simulink model "simulacia_zadanie"  (R2019b)
settings: Solver=VariableStepAuto  StartTime=0.0  StopTime=0.25  RelTol=1e-3
values from neighbouring files (symbols this model uses):
  B = 0    [poit8.m]
  J = 0.85e-04    (= 8.5e-05)    [poit8.m]
  Kp = 1/30*(3*pi*J*Td*w0^2-pi*B)    (= 0.0014835298642)    [poit8.m]
  s1 = serial('COM141','BaudRate', 9600)    [poit8.m]
  SetPoint = double(output)    [poit8.m]
  Ti = (30*Kp)/(pi*J*w0^3*Td)    (= 0.018)    [poit8.m]
  w1 = 1/Ti    (= 55.5555555556)    [poit8.m]
  w2 = 1000    [poit8.m]
  xi1 = 1    [poit8.m]
  xi2 = 1    [poit8.m]
libraries: simulink x1
settings Model: Creator=ChosenOneX  LastModifiedBy=ChosenOneX

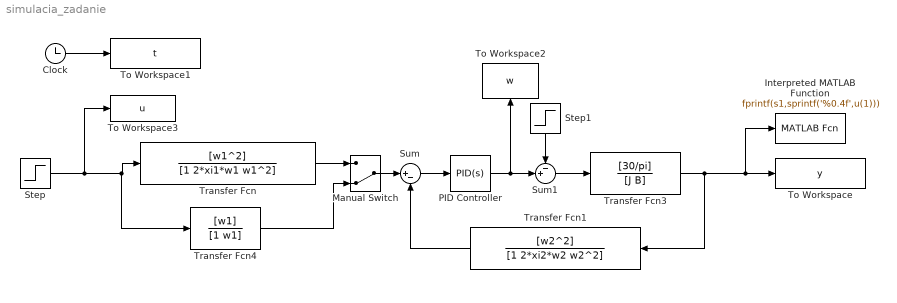
== system simulacia_zadanie ==
  Clock : Clock
  Interpreted MATLAB Function : MATLABFcn  MATLABFcn=fprintf(s1,sprintf('%0.4f',u(1)))  OutputDimensions=0
  Manual Switch : ManualSwitch  CurrentSetting=0
  PID Controller : simulink/Continuous/PID Controller  Controller=PID  Form=Parallel  TimeDomain=Continuous-time  SampleTime=-1  IntegratorMethod=Forward Euler  FilterMethod=Forward Euler  ControllerParametersSource=internal  P=Kp  I=Kp/Ti  D=0  UseFilter=on  N=100  TunerSelectOption=Transfer Function Based (PID Tuner App)  InitialConditionSource=internal  InitialConditionForIntegrator=0  InitialConditionForFilter=0  DifferentiatorICPrevScaledInput=0  ExternalReset=none  TrackingMode=off  Kt=1  LimitOutput=on  UpperSaturationLimit=7  LowerSaturationLimit=-7  LinearizeAsGain=on  AntiWindupMode=back-calculation  Kb=100  POutMin=[]  POutMax=[]  IOutMin=[]  IOutMax=[]  DOutMin=[]  DOutMax=[]  NOutMin=[]  NOutMax=[]  SumOutMin=[]  SumOutMax=[]  SaturationOutMin=[]  SaturationOutMax=[]  PParamMin=[]  PParamMax=[]  IParamMin=[]  IParamMax=[]  DParamMin=[]  DParamMax=[]  NParamMin=[]  NParamMax=[]  KbParamMin=[]  KbParamMax=[]  KtParamMin=[]  KtParamMax=[]  KbOutMin=[]  KbOutMax=[]  KtOutMin=[]  KtOutMax=[]  IntegratorOutMin=[]  IntegratorOutMax=[]  FilterOutMin=[]  FilterOutMax=[]  SumI1OutMin=[]  SumI1OutMax=[]  SumI2OutMin=[]  SumI2OutMax=[]  SumI3OutMin=[]  SumI3OutMax=[]  SumI4OutMin=[]  SumI4OutMax=[]  SumDOutMin=[]  SumDOutMax=[]  DifferentiatorOutMin=[]  DifferentiatorOutMax=[]  FilterDiffOutCoefMin=[]  FilterDiffOutCoefMax=[]  ReciprocalOutMin=[]  ReciprocalOutMax=[]  SumDenOutMin=[]  SumDenOutMax=[]  SumNumOutMin=[]  SumNumOutMax=[]  DivideOutMin=[]  DivideOutMax=[]  IntegratorContinuousStateAttributes=''  IntegratorStateMustResolveToSignalObject=off  IntegratorRTWStateStorageClass=Auto  FilterContinuousStateAttributes=''  FilterStateMustResolveToSignalObject=off  FilterRTWStateStorageClass=Auto  ParallelPVariant=InternalParameters  IdealPVariant=Disabled  IVariant=InternalParameters  DVariant=InternalParameters  IntegratorVariant=Continuous  SatVariant=Enabled  AWVariant=BackCalculation  PCopyVariant=Disabled  TRVariant=Disabled  FdbkBlocksVariant=Forward  IdealPFdbkVariant=Disabled  SatFdbkVariant=Disabled  DerivativeFilterVariant=ContFilter  NVariant=InternalParameters  NCopyVariant=Disabled  FilterICVariant=InternalICsFilter  IntegratorICVariant=InternalICs  ExternalResetVariant=Disabled  TRSumVariant=Passthrough  SumFdbkVariant=Disabled  SumVariant=Sum_PID
  Step : Step  Time=0  After=SetPoint*10  SampleTime=0
  Step1 : Step  Time=0.125  After=0.1  SampleTime=0
  Sum : Sum  Inputs=|+-
  Sum1 : Sum  Inputs=-+|
  To Workspace : ToWorkspace  VariableName=y  SampleTime=-1
  To Workspace1 : ToWorkspace  VariableName=t  SampleTime=-1
  To Workspace2 : ToWorkspace  VariableName=w  SampleTime=-1
  To Workspace3 : ToWorkspace  VariableName=u  SampleTime=-1
  Transfer Fcn : TransferFcn  Numerator=[w1^2]  Denominator=[1 2*xi1*w1 w1^2]
  Transfer Fcn1 : TransferFcn  Numerator=[w2^2]  Denominator=[1 2*xi2*w2 w2^2]
  Transfer Fcn3 : TransferFcn  Numerator=[30/pi]  Denominator=[J B]
  Transfer Fcn4 : TransferFcn  Numerator=[w1]  Denominator=[1 w1]
  wires:
  Transfer Fcn1/1 -> Sum/2
  Clock/1 -> To Workspace1/1
  Step/1 -> To Workspace3/1, Transfer Fcn4/1, Transfer Fcn/1
  Transfer Fcn4/1 -> Manual Switch/2
  Sum/1 -> PID Controller/1
  PID Controller/1 -> Sum1/2, To Workspace2/1
  Step1/1 -> Sum1/1
  Manual Switch/1 -> Sum/1
  Sum1/1 -> Transfer Fcn3/1
  Transfer Fcn/1 -> Manual Switch/1
  Transfer Fcn3/1 -> Interpreted MATLAB Function/1, To Workspace/1, Transfer Fcn1/1
